simulink model "IntModelY1_20212r"  (R2022b)
settings: Solver=VariableStepAuto  StartTime=0.0  StopTime=inf  RelTol=1e-3
model workspace (MAT data in the model file):
  firstWarning = 1
  originalScenarioChecksum = '114339432DE22364D47BB28FC96DC10C'
undefined symbols (not defined in the file or in its folder): Acceleration, ActorID, AngularVelocity, curvature, curvatureAhd, DefaultGear, DEND_B, DEND_S, DEND_T, direction, driving, gradbp, L, LF, LR, matlabshared, MAX_BRAKE, MAX_STEER, MAX_TORQUE, MCAR, MIN_BRAKE, MIN_STEER, MIN_TORQUE, NUMD_B, NUMD_S, NUMD_T, Pitch, Position, psi_o, R, Roll, RRdamp, SceneInfo, session, sigbuilder_block, STEER_RATIO, stopSign_ID, Tdead, thetaRefs, TL_ID, TrackWidth, Ts, ts, Vdead, Velocity, WB, X_o, xRef2s, Y_o, Yaw, yRef2s
libraries: drivingscenarioandsensors x8, simulink x3, drivingvehiclecontroller x2, trackingutilitieslib x2, robotalgslib x1, mpcadaslib x1, drivinglib x1, simulink_extras x1, autolibshared x1, vehdynlibviscommon x1, vehdynlibsteering x1
(part 2 of 3)

== system IntModelY1_20212r/Environment & Data/Sensors & Perception/Tracking ==
  Detections : Inport
  Camera : drivingscenarioandsensors/Vision Detection Generator  SensorIndex=1  DetectorOutput=Objects only  UpdateInterval=0.01  LaneUpdateInterval=0.1  SensorLocation=[1.9 0]  Height=1.1  Yaw=0  Pitch=1  Roll=0  BusNameSource=Auto  BusName=BusObjectDetections  BusName2Source=Auto  BusName2=BusLaneDetections  MaxNumDetectionsSource=Property  MaxNumDetections=10  MaxNumLanesSource=Property  MaxNumLanes=30  DetectionCoordinates=Ego Cartesian  SimulateUsing=Interpreted execution  MaxRange=150  BoundingBoxAccuracy=5  ProcessNoiseIntensity=5  MaxSpeed=100  MaxAllowedOcclusion=0.5  MinObjectImageSize=[2 2]  DetectionProbability=0.9  FalsePositivesPerImage=0.1  MinLaneImageSize=[20 3]  LaneBoundaryAccuracy=3  HasNoise=on  InitialSeedSource=Repeatable  InitialSeed=0  UsedSeed=0  ActorProfilesSource=From Scenario Reader block  ActorProfilesParameters=driving.internal.ActorProfilesParameters  ActorProfilesExpression=[struct('ActorID',1,'ClassID',1,'Length',4.7,'Width',1.8,'Height',1.4,'OriginOffset',[-1.35 0 0],'MeshVertices',[3.7 0.9 0.857439446366782;3.7 -0.9 0.857439446366782;3.7 -0.9 0.314878892733564;3.7 0.9 0.314878892733564;3.7 0.9 0.857439446366782;2.525 0.9 0.993079584775086;2.525 -0.9 0.993079584775086;3.7 -0.9 0.857439446366782;1.82 0.72 1.4;0.41 0.72 1.4;0.41 -0.72 1.4;1.82 -0.72 1.4;-0.295 0.9 0.993079584775086;-1 0.9 0.857439446366782;-1 -0.9 0.857439446366782;-0.295 -0.9 0.993079584775086;3.7 0.9 0.857439446366782;3.7 0.9 0.314878892733564;2.525 0.9 0.314878892733564;2.525 0.9 0.993079584775086;2.525 0.9 0.993079584775086;2.525 0.9 0.314878892733564;-0.295 0.9 0.314878892733564;-0.295 0.9 0.993079584775086;-0.295 0.9 0.993079584775086;-0.295 0.9 0.314878892733564;-1 0.9 0.355570934256055;-1 0.9 0.857439446366782;2.525 0.9 0.993079584775086;-0.295 0.9 0.993079584775086;0.41 0.72 1.4;1.82 0.72 1.4;3.7 -0.9 0.857439446366782;3.7 -0.9 0.314878892733564;2.525 -0.9 0.314878892733564;2.525 -0.9 0.993079584775086;2.525 -0.9 0.993079584775086;2.525 -0.9 0.314878892733564;-0.295 -0.9 0.314878892733564;-0.295 -0.9 0.993079584775086;-0.295 -0.9 0.993079584775086;-0.295 -0.9 0.314878892733564;-1 -0.9 0.355570934256055;-1 -0.9 0.857439446366782;2.525 -0.9 0.993079584775086;-0.295 -0.9 0.993079584775086;0.41 -0.72 1.4;1.82 -0.72 1.4;-0.295 0.9 0.993079584775086;-0.295 -0.9 0.993079584775086;0.41 -0.72 1.4;0.41 0.72 1.4;2.525 -0.9 0.993079584775086;1.82 -0.72 1.4;1.82 0.72 1.4;2.525 0.9 0.993079584775086;-1 0.9 0.857439446366782;-1 0.9 0.355570934256055;-1 -0.9 0.355570934256055;-1 -0.9 0.857439446366782;3.7 0.9 0.314878892733564;3.7 -0.9 0.314878892733564;-0.295 -0.9 0.314878892733564;-0.295 0.9 0.314878892733564;-0.295 0.9 0.314878892733564;-1 0.9 0.355570934256055;-1 -0.9 0.355570934256055;-0.295 -0.9 0.314878892733564;0 -0.63 0;0 -0.87 0;0.191030206995054 -0.63 0.0601365173421445;0.191030206995054 -0.87 0.0601365173421445;0.309093367795925 -0.63 0.217575963708927;0.309093367795925 -0.87 0.217575963708927;0.309093367795925 -0.63 0.412181821758201;0.309093367795925 -0.87 0.412181821758201;0.191030206995054 -0.63 0.569621268124983;0.191030206995054 -0.87 0.569621268124983;0 -0.63 0.629757785467128;0 -0.87 0.629757785467128;-0.191030206995054 -0.63 0.569621268124983;-0.191030206995054 -0.87 0.569621268124983;-0.309093367795925 -0.63 0.412181821758201;-0.309093367795925 -0.87 0.412181821758201;-0.309093367795925 -0.63 0.217575963708927;-0.309093367795925 -0.87 0.217575963708927;-0.191030206995054 -0.63 0.0601365173421445;-0.191030206995054 -0.87 0.0601365173421445;0 -0.63 0;0 -0.87 0;0 -0.63 0;0.191030206995054 -0.63 0.0601365173421445;0.309093367795925 -0.63 0.217575963708927;0.309093367795925 -0.63 0.412181821758201;0.191030206995054 -0.63 0.569621268124983;0 -0.63 0.629757785467128;-0.191030206995054 -0.63 0.569621268124983;-0.309093367795925 -0.63 0.412181821758201;-0.309093367795925 -0.63 0.217575963708927;-0.191030206995054 -0.63 0.0601365173421445;0 -0.87 0;0.191030206995054 -0.87 0.0601365173421445;0.309093367795925 -0.87 0.217575963708927;0.309093367795925 -0.87 0.412181821758201;0.191030206995054 -0.87 0.569621268124983;0 -0.87 0.629757785467128;-0.191030206995054 -0.87 0.569621268124983;-0.309093367795925 -0.87 0.412181821758201;-0.309093367795925 -0.87 0.217575963708927;-0.191030206995054 -0.87 0.0601365173421445;0 0.87 0;0 0.63 0;0.191030206995054 0.87 0.0601365173421445;0.191030206995054 0.63 0.0601365173421445;0.309093367795925 0.87 0.217575963708927;0.309093367795925 0.63 0.217575963708927;0.309093367795925 0.87 0.412181821758201;0.309093367795925 0.63 0.412181821758201;0.191030206995054 0.87 0.569621268124983;0.191030206995054 0.63 0.569621268124983;0 0.87 0.629757785467128;0 0.63 0.629757785467128;-0.191030206995054 0.87 0.569621268124983;-0.191030206995054 0.63 0.569621268124983;-0.309093367795925 0.87 0.412181821758201;-0.309093367795925 0.63 0.412181821758201;-0.309093367795925 0.87 0.217575963708927;-0.309093367795925 0.63 0.217575963708927;-0.191030206995054 0.87 0.0601365173421445;-0.191030206995054 0.63 0.0601365173421445;0 ...(+3718 chars)],'MeshFaces',[1 2 3;3 4 1;5 6 7;7 8 5;9 10 11;11 12 9;13 14 15;15 16 13;17 18 19;19 20 17;21 22 23;23 24 21;25 26 27;27 28 25;29 30 31;31 32 29;33 34 35;35 36 33;37 38 39;39 40 37;41 42 43;43 44 41;45 46 47;47 48 45;49 50 51;51 52 49;53 54 55;55 56 53;57 58 59;59 60 57;61 62 63;63 64 61;65 66 67;67 68 65;69 71 72;72 70 69;71 73 74;74 72 71;73 75 76;76 74 73;75 77 78;78 76 75;77 79 80;80 78 77;79 81 82;82 80 79;81 83 84;84 82 81;83 85 86;86 84 83;85 87 88;88 86 85;87 89 90;90 88 87;91 92 93;91 93 94;91 94 95;91 95 96;91 96 97;91 97 98;91 98 99;91 99 100;101 102 103;101 103 104;101 104 105;101 105 106;101 106 107;101 107 108;101 108 109;101 109 110;111 113 114;114 112 111;113 115 116;116 114 113;115 117 118;118 116 115;117 119 120;120 118 117;119 121 122;122 120 119;121 123 124;124 122 121;123 125 126;126 124 123;125 127 128;128 126 125;127 129 130;130 128 127;129 131 132;132 130 129;133 134 135;133 135 136;133 136 137;133 137 138;133 138 139;133 139 140;133 140 141;133 141 142;143 144 145;143 145 146;143 146 147;143 147 148;143 148 149;143 149 150;143 150 151;143 151 152;153 155 156;156 154 153;155 157 158;158 156 155;157 159 160;160 158 157;159 161 162;162 160 159;161 163 164;164 162 161;163 165 166;166 164 163;165 167 168;168 166 165;167 169 170;170 168 167;169 171 172;172 170 169;171 173 174;174 172 171;175 176 177;175 177 178;175 178 179;175 179 180;175 180 181;175 181 182;175 182 183;175 183 184;185 186 187;185 187 188;185 188 189;185 189 190;185 190 191;185 191 192;185 192 193;185 193 194;195 197 198;198 196 195;197 199 200;200 198 197;199 201 202;202 200 199;201 203 204;204 202 201;203 205 206;206 204 203;205 207 208;208 206 205;207 209 210;210 208 207;209 211 212;212 210 209;211 213 214;214 212 211;213 215 216;216 214 213;217 218 219;217 219 220;217 220 221;217 221 222;217 222 223;217 223 224;217 224 225;217 225 226;227 228 229;227 229 230;227 230 231;227 231 232;227 232 233;227 233 234;227 234 235;227 235 236],'RCSPattern',[10 10;10 10],'RCSAzimuthAngles',[-180 180],'RCSElevationAngles',[-90 90]); struct('ActorID',2,'ClassID',7,'Length',0.7,'Width',0.2,'Height',0.1,'OriginOffset',[0 0 0],'MeshVertices',[0.35 -0.1 0.1;0.35 0.1 0.1;-0.35 0.1 0.1;-0.35 -0.1 0.1;0.35 -0.1 0;0.35 0.1 0;-0.35 0.1 0;-0.35 -0.1 0],'MeshFaces',[6 2 1;1 5 6;8 4 3;3 7 8;6 7 3;3 2 6;5 1 4;4 8 5;4 1 2;2 3 4;7 6 5;5 8 7],'RCSPattern',[10 10;10 10],'RCSAzimuthAngles',[-180 180],'RCSElevationAngles',[-90 90])]  Intrinsics=driving.internal.cameraIntrinsics('FocalLength',[400 800],'PrincipalPoint',[320 240],'ImageSize',[480 640],'RadialDistortion',[0 0],'TangentialDistortion',[0 0],'Skew',0)
  Detection Concatenation : trackingutilitieslib/Detection Concatenation  NumInputs=2  BusNameSource=Property  BusName=Detections  SimulateUsing=Interpreted execution
  Multi-Object Tracker : drivinglib/Multi-Object Tracker  TrackerIndex=uint32( 0 )  FilterInitializationFcn=helperInitSimulinkDemoFilter  AssignmentThreshold=50  ConfirmationThreshold=[ 2, 3 ]  DeletionThreshold=[ 5, 5 ]  MaxNumTracks=20  MaxNumSensors=20  OOSMHandling=Neglect  StateParametersSimulink=struct  HasStateParametersInput=off  TimeInputSource=Auto  HasCostMatrixInput=off  HasDetectableTrackIDsInput=off  BusNameSource=Auto  BusName=BusMultiObjectTracker  TentativeTracksOutputPort=off  AllTracksOutputPort=off  SimulateUsing=Interpreted execution
  Radar Detection Generator : drivingscenarioandsensors/Radar Detection Generator  SensorIndex=2  UpdateInterval=0.01  SensorLocation=[ 1.5, 0 ]  Height=0.2  Yaw=0  Pitch=0  Roll=0  BusNameSource=Auto  BusName=BusRadarDetectionGenerator  MaxNumDetectionsSource=Property  MaxNumDetections=50  DetectionCoordinates=Ego Cartesian  SimulateUsing=Interpreted execution  AzimuthResolution=4  ElevationResolution=10  RangeResolution=2.5  RangeRateResolution=0.5  AzimuthBiasFraction=0.1  ElevationBiasFraction=0.1  RangeBiasFraction=0.05  RangeRateBiasFraction=0.05  FieldOfView=[ 60, 5 ]  MaxRange=150  RangeRateLimits=[ -100, 100 ]  DetectionProbability=0.9  FalseAlarmRate=1e-6  ReferenceRange=100  ReferenceRCS=0  HasElevation=off  HasRangeRate=on  HasNoise=on  HasFalseAlarms=on  HasOcclusion=on  InitialSeedSource=Repeatable  InitialSeed=0  UsedSeed=matlabshared.tracking.internal.SimulinkUtilities.seedManager(gcb)  ActorProfilesSource=Parameters  ActorProfilesParameters=driving.internal.ActorProfilesRadarParameters  ActorProfilesExpression=struct( 'ClassID', 0, 'Length', 4.7, 'Width', 1.8, 'Height', 1.4, 'OriginOffset', [ -1.35, 0, 0 ], 'RCSPattern', [ 10, 10; 10, 10 ], 'RCSAzimuthAngles', [ -180, 180 ], 'RCSElevationAngles', [ -90, 90 ] )
  Subsystem1 : Subsystem  Commented=on
  Confirmed_Tracks : Outport
  wires:
  Camera/1 -> Detection Concatenation/1  "Camera Detections"
  Radar Detection Generator/1 -> Detection Concatenation/2  "Lidar Detections"
  Detections/1 -> Radar Detection Generator/1, Camera/1
  Detection Concatenation/1 -> Multi-Object Tracker/1
  Multi-Object Tracker/1 -> Confirmed_Tracks/1

== system IntModelY1_20212r/Environment & Data/Visualisation & Data/Lights and Signs ID ==
  Constant : Constant  Value=TL_ID
  Constant1 : Constant  Value=stopSign_ID
  TL : Outport
  Stop_Sign : Outport  Port=2
  wires:
  Constant/1 -> TL/1
  Constant1/1 -> Stop_Sign/1

== system IntModelY1_20212r/Environment & Data/Visualisation & Data/Positions and States  ==
  note: Stop Sign positon
  note: Traffic Light Position and State
  <Actors> : Inport
  TL_id : Inport  Port=2
  ss_State : Inport  Port=3
  MATLAB Function1 : MATLAB Function  TreatAsAtomicUnit=on
  MATLAB Function2 : MATLAB Function  TreatAsAtomicUnit=on
  Traffic Light Sensor : Subsystem  mask{TrafficLightSensorModeSelection=Cycle}
      mask prompts: TrafficLightSensorModeSelection "Traffic Light Sensor Mode:"
      mask TypeOptions TrafficLightSensorModeSelection: Steady Green | Steady Red | Cycle
      mask DialogControl DescTextVar Prompt: Simulate a traffic light sensor.
  TL_poses : Outport
  ss_poses : Outport  Port=2
  wires:
  <Actors>/1 -> MATLAB Function2/1(Actors), MATLAB Function1/1(Actors)
  ss_State/1 -> MATLAB Function2/2(ss_State)
  TL_id/1 -> Traffic Light Sensor/1(TL_id)
  Traffic Light Sensor/1(TL_State) -> MATLAB Function1/2(TL_State)  "TL_State"
  MATLAB Function2/1(ss_poses) -> ss_poses/1
  MATLAB Function1/1(TL_poses) -> TL_poses/1

== system IntModelY1_20212r/Environment & Data/Visualisation & Data/Visualization ==
  note: Visualization
  TL1_poses : Inport
  Actors : Inport  Port=2
  EgoInfo : Inport  Port=3
  ss1_poses : Inport  Port=4
  Visualization : MATLABSystem  System=TL_vis
      mask Type: TL_vis
      mask Display:
      | disp('TL_vis');
      | port_label('input',1,'TL');
      | port_label('input',2,'TargetPoses');
      | port_label('input',3,'EgoInfo');
      | port_label('input',4,'SS');
  wires:
  EgoInfo/1 -> Visualization/3
  Actors/1 -> Visualization/2  "target_vehicle_poses"
  TL1_poses/1 -> Visualization/1
  ss1_poses/1 -> Visualization/4

== system IntModelY1_20212r/Reference Data/Theta/thetaBlocks ==
  note: theta calculated from Simulink blocks
  y : Inport
  x : Inport  Port=2
  dis : Inport  Port=3
  Atan2 : Trigonometry  Operator=atan2  ApproximationMethod=CORDIC
  Difference : simulink/Discrete/Difference  ICPrevInput=0.0  OutMin=[]  OutMax=[]  OutDataType=fixdt(1, 16)  OutScaling=2^-10  DoSatur=off
  Difference1 : simulink/Discrete/Difference  ICPrevInput=0.0  OutMin=[]  OutMax=[]  OutDataType=fixdt(1, 16)  OutScaling=2^-10  DoSatur=off
  IC : InitialCondition  Value=psi_o
  Radians to Degrees : simulink_extras/Transformations/Radians to Degrees
  Terminator : Terminator
  theta : Outport
  wires:
  IC/1 -> Radians to Degrees/1
  Atan2/1 -> IC/1
  dis/1 -> Terminator/1
  x/1 -> Difference1/1
  y/1 -> Difference/1
  Radians to Degrees/1 -> theta/1
  Difference/1 -> Atan2/1
  Difference1/1 -> Atan2/2

== system IntModelY1_20212r/Reference Data/Theta/thetaLt ==
  note: Check out the script "setUpModel" to understand how we have calculated theta
  note: theta based on lookup table
  y : Inport
  x : Inport  Port=2
  dis : Inport  Port=3
  Terminator : Terminator
  Terminator1 : Terminator
  Theta Ref : Lookup_n-D  NumberOfTableDimensions=1  BreakpointsForDimension1=gradbp  Table=thetaRefs  InternalRulePriority=Speed  RndMeth=Simplest
  theta : Outport
  wires:
  Theta Ref/1 -> theta/1
  dis/1 -> Theta Ref/1
  x/1 -> Terminator1/1
  y/1 -> Terminator/1

== system IntModelY1_20212r/Vehicle Dynamics/Subsystem/Signal Builder ==
  Demux : Demux  Tag=STV Demux  Outputs=3
      settings: DisplayOption=none
  FromWs : FromWorkspace  Tag=STV FromWs  VariableName=tuvar
      SigBuilderData=|
      | common.afterFinalStr = 'Extrapolate'
      | common.sampleTime = 0
      | dataSet.timeRange = [0 3.5]
      | dataSet.name = 'DriveAndTurn'
      | sbobj.Groups.Name = 'DriveAndTurn'
      | sbobj.Groups.Signals(1).Name = 'Normalized Torque'
      | sbobj.Groups.Signals(1).XData = [0 1 1 2 2 3.5]
      | sbobj.Groups.Signals(1).YData = [1 1 0 0 1 1]
      | sbobj.Groups.Signals(2).Name = 'Normalized Brake'
      | sbobj.Groups.Signals(2).XData = [0 1 1 2 2 3.5]
      | sbobj.Groups.Signals(2).YData = [0 0 1 1 0 0]
      | sbobj.Groups.Signals(3).Name = 'Normalized Steer'
      | sbobj.Groups.Signals(3).XData = [0 0.5 0.6 1.02 1.02 2 2.5 3 3.5]
      | sbobj.Groups.Signals(3).YData = [-0.02 -0.02 -0.02 -0.3 -1.02 -0.92 -0.34 0.14 0.22]
      | sbobj.Groups.TimeRange = [0 3.5]
  Normalized Torque : Outport  Tag=STV Outport
  Normalized Brake : Outport  Tag=STV Outport  Port=2
  Normalized Steer : Outport  Tag=STV Outport  Port=3
  wires:
  FromWs/1 -> Demux/1
  Demux/1 -> Normalized Torque/1
  Demux/2 -> Normalized Brake/1
  Demux/3 -> Normalized Steer/1

== system IntModelY1_20212r/Vehicle Dynamics/VehicleDynamics/Vehicle XY Plotter ==
  VehFdbk : Inport
  VehFdbk1 : Inport  Port=2
  Bus Selector1 : BusSelector  OutputSignals=InertFrm.Cg.Ang.phi,InertFrm.Cg.Ang.theta,InertFrm.Cg.Ang.psi  OutputAsBus=on
  Bus Selector3 : BusSelector  OutputSignals=InertFrm.Geom.Disp.X,InertFrm.Geom.Disp.Y,InertFrm.Geom.Disp.Z  OutputAsBus=on
  Bus Selector4 : BusSelector  OutputSignals=InertFrm.Cg.Vel.Xdot,InertFrm.Cg.Vel.Ydot  OutputAsBus=on
  Bus to Vector : BusToVector
  Bus to Vector1 : BusToVector
  Bus to Vector2 : BusToVector
  Constant4 : Constant  Value=0
  Ground : Ground
  Rate Transition{1..2,5..6} (4 alike) : RateTransition  OutPortSampleTime=pltDT
  Vector Concatenate : Concatenate
  Vector Concatenate1 : Concatenate  NumInputs=4
  Vehicle XY Plotter : vehdynlibviscommon/Vehicle XY Plotter  w=w  a=a  b=b  figBorder=2000  bufferSize=bufferSize  extStats=off  extTireF=off
  wires:
  Bus to Vector2/1 -> Rate Transition1/1  "InertCGDisp"
  Rate Transition5/1 -> Vehicle XY Plotter/1
  Bus Selector4/1 -> Bus to Vector1/1
  Rate Transition1/1 -> Vehicle XY Plotter/2
  Rate Transition6/1 -> Vehicle XY Plotter/3
  Vector Concatenate/1 -> Rate Transition6/1  "InertCGVel"
  Bus Selector1/1 -> Bus to Vector2/1
  Bus to Vector/1 -> Rate Transition5/1  "InertCGDisp"
  Bus Selector3/1 -> Bus to Vector/1
  Bus to Vector1/1 -> Vector Concatenate/1
  Ground/1 -> Vector Concatenate/2
  VehFdbk/1 -> Bus Selector1/1, Bus Selector4/1, Bus Selector3/1
  Rate Transition2/1 -> Vehicle XY Plotter/4
  Constant4/1 -> Vector Concatenate1/4, Vector Concatenate1/3
  VehFdbk1/1 -> Vector Concatenate1/2, Vector Concatenate1/1  "delta"
  Vector Concatenate1/1 -> Rate Transition2/1  "delta"

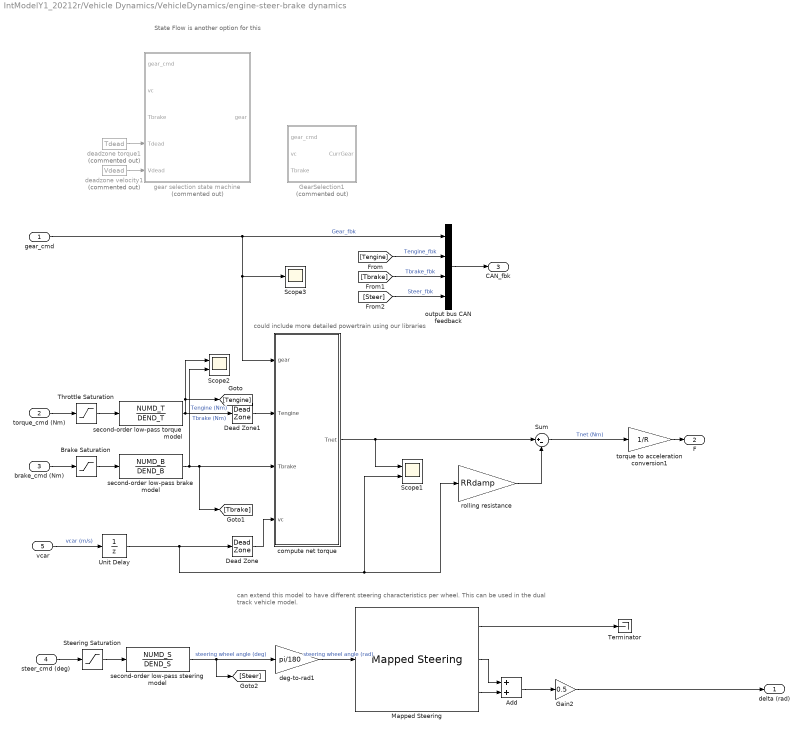
== system IntModelY1_20212r/Vehicle Dynamics/VehicleDynamics/engine-steer-brake dynamics ==
  note: State Flow is another option for this
  note: could include more detailed powertrain using our libraries
  note: can extend this model to have different steering characteristics per wheel. This can be used in the dual track vehicle model.
  gear_cmd : Inport
  torque_cmd (Nm) : Inport  Port=2
  brake_cmd (Nm) : Inport  Port=3
  steer_cmd (deg) : Inport  Port=4
  vcar : Inport  Port=5
  Add : Sum
  Brake Saturation : Saturate  UpperLimit=MAX_BRAKE  LowerLimit=MIN_BRAKE
  Dead Zone : DeadZone  LowerValue=-Vdead  UpperValue=Vdead
  Dead Zone1 : DeadZone  LowerValue=-Tdead  UpperValue=Tdead
  Gain2 : Gain  Gain=0.5
  GearSelection1 : Stateflow chart  Commented=on  TreatAsAtomicUnit=on  SystemSampleTime=ts
      settings: PortSchema="{\"entries\":[{\"content\":{\"sides\":[{\"content\":{\"connectorIds\":[\"In3\",\"In2\",\"In1\"]},\"type\":\"ConnectorPlacement.EquallySpacedRectSide\",\"uuid\":\"465e5722-891f-481b-b3b6-2b8339e8e743\"},{\"content\":{\"connectorIds\":[\"Out1\"],\"side\":\"RIGHT\"},\"type\":\"ConnectorPlacement.EquallySpacedRectSide\",\"uuid\":\"28ef13cd-41d9-4e2e-8cd9-9157abf573a9\"},{\"content\":{\"connectorIds\":[],\"side\":\"TOP\"},\"type\":\"ConnectorPlacement.EquallySpacedRectSide\",\"uuid\":\"44f19923-60ae-466f-ad2a-756f1033b52e\"},{\"content\":{\"connectorIds\":[],\"side\":\"HIDDEN\"},\"type\":\"ConnectorPlacement.EquallySpacedRectSide\",\"uuid\":\"d5a146f0-4328-42be-94e3-09f51634e7da\"}]},\"type\":\"ConnectorPlacement.EquallySpacedConnector\",\"uuid\":\"14e271af-3da2-4f7d-9688-fcc3c9792006\"}],\"packageUris\":[\"http://schema.mathworks.com/mf0/Connector/R2020b\"],\"version\":\"1.0\"}"
  Mapped Steering : vehdynlibsteering/Mapped Steering  SpdDpd=off  IndexType=Steering wheel angle  GrType=Constant  StrgAngBpts=[-1.5*pi 1.5*pi]  RackDispBpts=[-40 -19.2 -4.53 4.53 19.2 40]  Gr=8.28*2*pi  GrTbl=[9.87 9.87 7.16 7.16 9.87 9.87]*2*pi  WhlLftTbl=[-1.5*pi 1.5*pi]*STEER_RATIO  WhlRghtTbl=[-1.5*pi 1.5*pi]*STEER_RATIO  VehSpdBpts=[-1 1]  SpdFctTbl=[1 1]  aMode=2
  Scope1 : Scope  NumInputPorts=2
  Scope2 : Scope  NumInputPorts=2
  Scope3 : Scope
  Steering Saturation : Saturate  UpperLimit=MAX_STEER  LowerLimit=MIN_STEER
  Sum : Sum  Inputs=|+-
  Terminator : Terminator
  Throttle Saturation : Saturate  UpperLimit=MAX_TORQUE  LowerLimit=MIN_TORQUE
  Unit Delay : UnitDelay  SampleTime=-1  HasFrameUpgradeWarning=on
  compute net torque : MATLAB Function  TreatAsAtomicUnit=on  SystemSampleTime=ts
  deadzone torque1 : Constant  Commented=on  Value=Tdead  SampleTime=ts
  deadzone velocity1 : Constant  Commented=on  Value=Vdead  SampleTime=ts
  deg-to-rad1 : Gain  Gain=pi/180
  gear selection state machine : MATLAB Function  Commented=on  TreatAsAtomicUnit=on  SystemSampleTime=ts
  output bus CAN feedback : BusCreator  Inputs=4
  rolling resistance : Gain  Gain=RRdamp
  second-order low-pass brake model : DiscreteTransferFcn  Numerator=NUMD_B  Denominator=DEND_B  SampleTime=ts
  second-order low-pass steering model : DiscreteTransferFcn  Numerator=NUMD_S  Denominator=DEND_S  SampleTime=ts
  second-order low-pass torque model : DiscreteTransferFcn  Numerator=NUMD_T  Denominator=DEND_T  SampleTime=ts
  torque to acceleration conversion1 : Gain  Gain=1/R
  delta (rad) : Outport  VectorParamsAs1DForOutWhenUnconnected=off
  F : Outport  Port=2  VectorParamsAs1DForOutWhenUnconnected=off
  CAN_fbk : Outport  Port=3  VectorParamsAs1DForOutWhenUnconnected=off
  wires:
  steer_cmd (deg)/1 -> Steering Saturation/1
  torque_cmd (Nm)/1 -> Throttle Saturation/1
  brake_cmd (Nm)/1 -> Brake Saturation/1
  second-order low-pass steering model/1 -> deg-to-rad1/1, [Steer]  "steering wheel angle (deg)"
  Throttle Saturation/1 -> second-order low-pass torque model/1
  Brake Saturation/1 -> second-order low-pass brake model/1
  Steering Saturation/1 -> second-order low-pass steering model/1
  vcar/1 -> Unit Delay/1  "vcar (m/s)"
  second-order low-pass brake model/1 -> [Tbrake], compute net torque/3(Tbrake), Scope2/2  "Tbrake (Nm)"
  second-order low-pass torque model/1 -> Dead Zone1/1, [Tengine], Scope2/1  "Tengine (Nm)"
  compute net torque/1(Tnet) -> Scope1/1, Sum/1
  rolling resistance/1 -> Sum/2
  deadzone velocity1/1 -> gear selection state machine/5(Vdead)
  deadzone torque1/1 -> gear selection state machine/4(Tdead)
  gear_cmd/1 -> output bus CAN feedback/1, Scope3/1, compute net torque/1(gear)  "Gear_fbk"
  output bus CAN feedback/1 -> CAN_fbk/1
  [Tengine] -> output bus CAN feedback/2  "Tengine_fbk"
  [Tbrake] -> output bus CAN feedback/3  "Tbrake_fbk"
  [Steer] -> output bus CAN feedback/4  "Steer_fbk"
  Mapped Steering/2 -> Add/1
  Mapped Steering/3 -> Add/2
  Add/1 -> Gain2/1
  torque to acceleration conversion1/1 -> F/1
  Mapped Steering/1 -> Terminator/1
  deg-to-rad1/1 -> Mapped Steering/1  "steering wheel angle (rad)"
  Sum/1 -> torque to acceleration conversion1/1  "Tnet (Nm)"
  Dead Zone/1 -> compute net torque/4(vc)
  Dead Zone1/1 -> compute net torque/2(Tengine)
  Unit Delay/1 -> Scope1/2, rolling resistance/1, Dead Zone/1
  Gain2/1 -> delta (rad)/1

== system IntModelY1_20212r/Controllers/Lateral Controllers/Pure Pursuit Controller1/Wheel Steering Angle Formulation ==
  alpha : Inport
  Bicycle length : Constant  Value=L
  Constant : Constant  Value=2
  Divide : Product  Inputs=*/
  Lookahead distance : Constant  Value=ld
  Product : Product
  Product1 : Product
  Sine Wave : Sin  TimeSource=Use external signal  SampleTime=0
  Trigonometric Function : Trigonometry  Operator=atan
  Al : Outport
  wires:
  Sine Wave/1 -> Product1/2
  Bicycle length/1 -> Product/2
  Constant/1 -> Product/1
  Product1/1 -> Divide/1
  Product/1 -> Product1/1
  Divide/1 -> Trigonometric Function/1
  Trigonometric Function/1 -> Al/1
  alpha/1 -> Sine Wave/1
  Lookahead distance/1 -> Divide/2

== system IntModelY1_20212r/Controllers/Subsystem3/Subsystem1/Subsystem2 ==
  acc_cmd : Inport
  decc_cmd : Inport  Port=2
  Subsystem : Subsystem
  Subsystem1 : Subsystem
  T_eng_cmd : Outport
  brake_cmd : Outport  Port=2
  wires:
  acc_cmd/1 -> Subsystem/1(acc_cmd)
  Subsystem/1(T_eng_cmd) -> T_eng_cmd/1
  decc_cmd/1 -> Subsystem1/1(decc_cmd)
  Subsystem1/1(T_brake_cmd) -> brake_cmd/1

== system IntModelY1_20212r/Controllers/Subsystem3/Subsystem2/Subsystem2 ==
  acc_cmd : Inport
  decc_cmd : Inport  Port=2
  Subsystem : Subsystem
  Subsystem1 : Subsystem
  T_eng_cmd : Outport
  brake_cmd : Outport  Port=2
  wires:
  acc_cmd/1 -> Subsystem/1(acc_cmd)
  Subsystem/1(T_eng_cmd) -> T_eng_cmd/1
  decc_cmd/1 -> Subsystem1/1(decc_cmd)
  Subsystem1/1(T_brake_cmd) -> brake_cmd/1

== system IntModelY1_20212r/Environment & Data/Sensors & Perception/Tracking/Subsystem1 ==
  In2 : Inport
  EgoV : Inport  Port=2
  Camera : drivingscenarioandsensors/Vision Detection Generator  SensorIndex=1  DetectorOutput=Objects only  UpdateInterval=0.1  LaneUpdateInterval=0.1  SensorLocation=[1.9 0]  Height=1.1  Yaw=0  Pitch=1  Roll=0  BusNameSource=Auto  BusName=BusObjectDetections  BusName2Source=Auto  BusName2=BusLaneDetections  MaxNumDetectionsSource=Property  MaxNumDetections=10  MaxNumLanesSource=Property  MaxNumLanes=30  DetectionCoordinates=Ego Cartesian  SimulateUsing=Interpreted execution  MaxRange=150  BoundingBoxAccuracy=5  ProcessNoiseIntensity=5  MaxSpeed=100  MaxAllowedOcclusion=0.5  MinObjectImageSize=[5 5]  DetectionProbability=0.9  FalsePositivesPerImage=0.1  MinLaneImageSize=[20 3]  LaneBoundaryAccuracy=3  HasNoise=on  InitialSeedSource=Repeatable  InitialSeed=0  UsedSeed=0  ActorProfilesSource=From Scenario Reader block  ActorProfilesParameters=driving.internal.ActorProfilesParameters  ActorProfilesExpression=[struct('ActorID',1,'ClassID',1,'Length',4.7,'Width',1.8,'Height',1.4,'OriginOffset',[-1.35 0 0],'MeshVertices',[3.7 0.9 0.857439446366782;3.7 -0.9 0.857439446366782;3.7 -0.9 0.314878892733564;3.7 0.9 0.314878892733564;3.7 0.9 0.857439446366782;2.525 0.9 0.993079584775086;2.525 -0.9 0.993079584775086;3.7 -0.9 0.857439446366782;1.82 0.72 1.4;0.41 0.72 1.4;0.41 -0.72 1.4;1.82 -0.72 1.4;-0.295 0.9 0.993079584775086;-1 0.9 0.857439446366782;-1 -0.9 0.857439446366782;-0.295 -0.9 0.993079584775086;3.7 0.9 0.857439446366782;3.7 0.9 0.314878892733564;2.525 0.9 0.314878892733564;2.525 0.9 0.993079584775086;2.525 0.9 0.993079584775086;2.525 0.9 0.314878892733564;-0.295 0.9 0.314878892733564;-0.295 0.9 0.993079584775086;-0.295 0.9 0.993079584775086;-0.295 0.9 0.314878892733564;-1 0.9 0.355570934256055;-1 0.9 0.857439446366782;2.525 0.9 0.993079584775086;-0.295 0.9 0.993079584775086;0.41 0.72 1.4;1.82 0.72 1.4;3.7 -0.9 0.857439446366782;3.7 -0.9 0.314878892733564;2.525 -0.9 0.314878892733564;2.525 -0.9 0.993079584775086;2.525 -0.9 0.993079584775086;2.525 -0.9 0.314878892733564;-0.295 -0.9 0.314878892733564;-0.295 -0.9 0.993079584775086;-0.295 -0.9 0.993079584775086;-0.295 -0.9 0.314878892733564;-1 -0.9 0.355570934256055;-1 -0.9 0.857439446366782;2.525 -0.9 0.993079584775086;-0.295 -0.9 0.993079584775086;0.41 -0.72 1.4;1.82 -0.72 1.4;-0.295 0.9 0.993079584775086;-0.295 -0.9 0.993079584775086;0.41 -0.72 1.4;0.41 0.72 1.4;2.525 -0.9 0.993079584775086;1.82 -0.72 1.4;1.82 0.72 1.4;2.525 0.9 0.993079584775086;-1 0.9 0.857439446366782;-1 0.9 0.355570934256055;-1 -0.9 0.355570934256055;-1 -0.9 0.857439446366782;3.7 0.9 0.314878892733564;3.7 -0.9 0.314878892733564;-0.295 -0.9 0.314878892733564;-0.295 0.9 0.314878892733564;-0.295 0.9 0.314878892733564;-1 0.9 0.355570934256055;-1 -0.9 0.355570934256055;-0.295 -0.9 0.314878892733564;0 -0.63 0;0 -0.87 0;0.191030206995054 -0.63 0.0601365173421445;0.191030206995054 -0.87 0.0601365173421445;0.309093367795925 -0.63 0.217575963708927;0.309093367795925 -0.87 0.217575963708927;0.309093367795925 -0.63 0.412181821758201;0.309093367795925 -0.87 0.412181821758201;0.191030206995054 -0.63 0.569621268124983;0.191030206995054 -0.87 0.569621268124983;0 -0.63 0.629757785467128;0 -0.87 0.629757785467128;-0.191030206995054 -0.63 0.569621268124983;-0.191030206995054 -0.87 0.569621268124983;-0.309093367795925 -0.63 0.412181821758201;-0.309093367795925 -0.87 0.412181821758201;-0.309093367795925 -0.63 0.217575963708927;-0.309093367795925 -0.87 0.217575963708927;-0.191030206995054 -0.63 0.0601365173421445;-0.191030206995054 -0.87 0.0601365173421445;0 -0.63 0;0 -0.87 0;0 -0.63 0;0.191030206995054 -0.63 0.0601365173421445;0.309093367795925 -0.63 0.217575963708927;0.309093367795925 -0.63 0.412181821758201;0.191030206995054 -0.63 0.569621268124983;0 -0.63 0.629757785467128;-0.191030206995054 -0.63 0.569621268124983;-0.309093367795925 -0.63 0.412181821758201;-0.309093367795925 -0.63 0.217575963708927;-0.191030206995054 -0.63 0.0601365173421445;0 -0.87 0;0.191030206995054 -0.87 0.0601365173421445;0.309093367795925 -0.87 0.217575963708927;0.309093367795925 -0.87 0.412181821758201;0.191030206995054 -0.87 0.569621268124983;0 -0.87 0.629757785467128;-0.191030206995054 -0.87 0.569621268124983;-0.309093367795925 -0.87 0.412181821758201;-0.309093367795925 -0.87 0.217575963708927;-0.191030206995054 -0.87 0.0601365173421445;0 0.87 0;0 0.63 0;0.191030206995054 0.87 0.0601365173421445;0.191030206995054 0.63 0.0601365173421445;0.309093367795925 0.87 0.217575963708927;0.309093367795925 0.63 0.217575963708927;0.309093367795925 0.87 0.412181821758201;0.309093367795925 0.63 0.412181821758201;0.191030206995054 0.87 0.569621268124983;0.191030206995054 0.63 0.569621268124983;0 0.87 0.629757785467128;0 0.63 0.629757785467128;-0.191030206995054 0.87 0.569621268124983;-0.191030206995054 0.63 0.569621268124983;-0.309093367795925 0.87 0.412181821758201;-0.309093367795925 0.63 0.412181821758201;-0.309093367795925 0.87 0.217575963708927;-0.309093367795925 0.63 0.217575963708927;-0.191030206995054 0.87 0.0601365173421445;-0.191030206995054 0.63 0.0601365173421445;0 ...(+3718 chars)],'MeshFaces',[1 2 3;3 4 1;5 6 7;7 8 5;9 10 11;11 12 9;13 14 15;15 16 13;17 18 19;19 20 17;21 22 23;23 24 21;25 26 27;27 28 25;29 30 31;31 32 29;33 34 35;35 36 33;37 38 39;39 40 37;41 42 43;43 44 41;45 46 47;47 48 45;49 50 51;51 52 49;53 54 55;55 56 53;57 58 59;59 60 57;61 62 63;63 64 61;65 66 67;67 68 65;69 71 72;72 70 69;71 73 74;74 72 71;73 75 76;76 74 73;75 77 78;78 76 75;77 79 80;80 78 77;79 81 82;82 80 79;81 83 84;84 82 81;83 85 86;86 84 83;85 87 88;88 86 85;87 89 90;90 88 87;91 92 93;91 93 94;91 94 95;91 95 96;91 96 97;91 97 98;91 98 99;91 99 100;101 102 103;101 103 104;101 104 105;101 105 106;101 106 107;101 107 108;101 108 109;101 109 110;111 113 114;114 112 111;113 115 116;116 114 113;115 117 118;118 116 115;117 119 120;120 118 117;119 121 122;122 120 119;121 123 124;124 122 121;123 125 126;126 124 123;125 127 128;128 126 125;127 129 130;130 128 127;129 131 132;132 130 129;133 134 135;133 135 136;133 136 137;133 137 138;133 138 139;133 139 140;133 140 141;133 141 142;143 144 145;143 145 146;143 146 147;143 147 148;143 148 149;143 149 150;143 150 151;143 151 152;153 155 156;156 154 153;155 157 158;158 156 155;157 159 160;160 158 157;159 161 162;162 160 159;161 163 164;164 162 161;163 165 166;166 164 163;165 167 168;168 166 165;167 169 170;170 168 167;169 171 172;172 170 169;171 173 174;174 172 171;175 176 177;175 177 178;175 178 179;175 179 180;175 180 181;175 181 182;175 182 183;175 183 184;185 186 187;185 187 188;185 188 189;185 189 190;185 190 191;185 191 192;185 192 193;185 193 194;195 197 198;198 196 195;197 199 200;200 198 197;199 201 202;202 200 199;201 203 204;204 202 201;203 205 206;206 204 203;205 207 208;208 206 205;207 209 210;210 208 207;209 211 212;212 210 209;211 213 214;214 212 211;213 215 216;216 214 213;217 218 219;217 219 220;217 220 221;217 221 222;217 222 223;217 223 224;217 224 225;217 225 226;227 228 229;227 229 230;227 230 231;227 231 232;227 232 233;227 233 234;227 234 235;227 235 236],'RCSPattern',[10 10;10 10],'RCSAzimuthAngles',[-180 180],'RCSElevationAngles',[-90 90]); struct('ActorID',2,'ClassID',7,'Length',0.7,'Width',0.2,'Height',0.1,'OriginOffset',[0 0 0],'MeshVertices',[0.35 -0.1 0.1;0.35 0.1 0.1;-0.35 0.1 0.1;-0.35 -0.1 0.1;0.35 -0.1 0;0.35 0.1 0;-0.35 0.1 0;-0.35 -0.1 0],'MeshFaces',[6 2 1;1 5 6;8 4 3;3 7 8;6 7 3;3 2 6;5 1 4;4 8 5;4 1 2;2 3 4;7 6 5;5 8 7],'RCSPattern',[10 10;10 10],'RCSAzimuthAngles',[-180 180],'RCSElevationAngles',[-90 90])]  Intrinsics=driving.internal.cameraIntrinsics('FocalLength',[800 800],'PrincipalPoint',[320 240],'ImageSize',[480 640],'RadialDistortion',[0 0],'TangentialDistortion',[0 0],'Skew',0)
  Detection Concatenation : trackingutilitieslib/Detection Concatenation  NumInputs=3  BusNameSource=Auto  BusName=BusDetectionConcatenation  SimulateUsing=Interpreted execution
  Lidar Point Cloud Generator : drivingscenarioandsensors/Lidar Point Cloud Generator  SensorIndex=2  UpdateInterval=0.1  SensorLocation=[1.5 0]  Height=1.6  Yaw=0  Pitch=0  Roll=0  DetectionCoordinates=Ego Cartesian  HasEgoVehicle=on  EgoVehicleActorID=1  HasRoadsInputPort=on  ActorProfilesSource=From Scenario Reader block  ActorProfilesVariableName=actor_profiles  MaxRange=120  RangeAccuracy=0.002  AzimuthResolution=0.16  ElevationResolution=1.25  AzimuthLimits=[-60 60]  ElevationLimits=[ -20, 20 ]  HasNoise=on
  Lidar Point Cloud Generator1 : drivingscenarioandsensors/Lidar Point Cloud Generator  SensorIndex=3  UpdateInterval=0.1  SensorLocation=[1.5 0]  Height=1.6  Yaw=0  Pitch=0  Roll=0  DetectionCoordinates=Ego Cartesian  HasEgoVehicle=on  EgoVehicleActorID=1  HasRoadsInputPort=on  ActorProfilesSource=From Scenario Reader block  ActorProfilesVariableName=actor_profiles  MaxRange=120  RangeAccuracy=0.002  AzimuthResolution=0.16  ElevationResolution=1.25  AzimuthLimits=[60 180]  ElevationLimits=[ -20, 20 ]  HasNoise=on
  Lidar Point Cloud Generator2 : drivingscenarioandsensors/Lidar Point Cloud Generator  SensorIndex=4  UpdateInterval=0.1  SensorLocation=[1.5 0]  Height=1.6  Yaw=0  Pitch=0  Roll=0  DetectionCoordinates=Ego Cartesian  HasEgoVehicle=on  EgoVehicleActorID=1  HasRoadsInputPort=on  ActorProfilesSource=From Scenario Reader block  ActorProfilesVariableName=actor_profiles  MaxRange=120  RangeAccuracy=0.002  AzimuthResolution=0.16  ElevationResolution=1.25  AzimuthLimits=[-180 -60]  ElevationLimits=[ -20, 20 ]  HasNoise=on
  Camera Detections : Outport
  Radar detections : Outport  Port=2
  wires:
  EgoV/1 -> Lidar Point Cloud Generator1/2, Lidar Point Cloud Generator/2, Lidar Point Cloud Generator2/2
  Lidar Point Cloud Generator1/1 -> Detection Concatenation/2  "Lidar Detections"
  Lidar Point Cloud Generator2/1 -> Detection Concatenation/3  "Lidar Detections"
  Detection Concatenation/1 -> Radar detections/1
  Camera/1 -> Camera Detections/1  "Camera Detections"
  In2/1 -> Camera/1, Lidar Point Cloud Generator/1, Lidar Point Cloud Generator1/1, Lidar Point Cloud Generator2/1
  Lidar Point Cloud Generator/1 -> Detection Concatenation/1  "Lidar Detections"

== system IntModelY1_20212r/Environment & Data/Visualisation & Data/Positions and States /Traffic Light Sensor ==
  note: Traffic Light Sensor
  TL_id : Inport
  Bus Creator : BusCreator  Inputs=2
  LightConfiguration : Constant  Value=TrafficLightSensorModeSelection
  Traffic Light Switching Logic : Stateflow chart  TreatAsAtomicUnit=on
  TL_State : Outport
  wires:
  LightConfiguration/1 -> Traffic Light Switching Logic/1(LightConfig)
  TL_id/1 -> Traffic Light Switching Logic/2(TL_id)
  Bus Creator/1 -> TL_State/1
  Traffic Light Switching Logic/2(trafficLight) -> Bus Creator/1
  Traffic Light Switching Logic/1(TL_ID) -> Bus Creator/2

== system IntModelY1_20212r/Controllers/Subsystem3/Subsystem1/Subsystem2/Subsystem ==
  acc_cmd : Inport
  Constant1 : Constant  Value=MCAR
  Gain : Gain  Gain=1.1*MCAR
  Gain1 : Gain  Gain=1.2*0.3*2/2
  Gain2 : Gain  Gain=0.7*9.81
  Gain4 : Gain  Gain=R/(7.05*0.8)
  Integrator : Integrator  ExternalReset=falling
  Square : Math  Operator=square
  Sum : Sum  Inputs=+++
  T_eng_cmd : Outport
  wires:
  Constant1/1 -> Gain2/1
  Gain/1 -> Sum/3
  Sum/1 -> Gain4/1
  acc_cmd/1 -> Gain/1, Integrator/2, Integrator/1
  Gain2/1 -> Sum/2
  Gain1/1 -> Sum/1  "F_aero"
  Gain4/1 -> T_eng_cmd/1  "T_eng"
  Integrator/1 -> Square/1  "v"
  Square/1 -> Gain1/1

== system IntModelY1_20212r/Controllers/Subsystem3/Subsystem1/Subsystem2/Subsystem1 ==
  decc_cmd : Inport
  Constant1 : Constant  Value=MCAR
  Gain : Gain  Gain=1.1*MCAR
  Gain1 : Gain  Gain=1.2*0.3*2/2
  Gain2 : Gain  Gain=0.7*9.81
  Gain4 : Gain  Gain=-R/(7.05*0.8)
  Integrator : Integrator  ExternalReset=falling
  Square : Math  Operator=square
  Sum : Sum  Inputs=+++
  T_brake_cmd : Outport
  wires:
  Square/1 -> Gain1/1
  Integrator/1 -> Square/1  "v"
  Gain4/1 -> T_brake_cmd/1  "T_eng"
  Gain1/1 -> Sum/1  "F_aero"
  Gain2/1 -> Sum/2
  decc_cmd/1 -> Integrator/2, Integrator/1, Gain/1
  Sum/1 -> Gain4/1
  Gain/1 -> Sum/3
  Constant1/1 -> Gain2/1

== system IntModelY1_20212r/Controllers/Subsystem3/Subsystem2/Subsystem2/Subsystem ==
  acc_cmd : Inport
  Constant1 : Constant  Value=MCAR
  Gain : Gain  Gain=1.1*MCAR
  Gain1 : Gain  Gain=1.2*0.3*2/2
  Gain2 : Gain  Gain=0.7*9.81
  Gain4 : Gain  Gain=R/(7.05*0.8)
  Integrator : Integrator  ExternalReset=falling
  Square : Math  Operator=square
  Sum : Sum  Inputs=+++
  T_eng_cmd : Outport
  wires:
  Constant1/1 -> Gain2/1
  Gain/1 -> Sum/3
  Sum/1 -> Gain4/1
  acc_cmd/1 -> Gain/1, Integrator/2, Integrator/1
  Gain2/1 -> Sum/2
  Gain1/1 -> Sum/1  "F_aero"
  Gain4/1 -> T_eng_cmd/1  "T_eng"
  Integrator/1 -> Square/1  "v"
  Square/1 -> Gain1/1

== system IntModelY1_20212r/Controllers/Subsystem3/Subsystem2/Subsystem2/Subsystem1 ==
  decc_cmd : Inport
  Constant1 : Constant  Value=MCAR
  Gain : Gain  Gain=1.1*MCAR
  Gain1 : Gain  Gain=1.2*0.3*2/2
  Gain2 : Gain  Gain=0.7*9.81
  Gain4 : Gain  Gain=-R/(7.05*0.8)
  Integrator : Integrator  ExternalReset=falling
  Square : Math  Operator=square
  Sum : Sum  Inputs=+++
  T_brake_cmd : Outport
  wires:
  Square/1 -> Gain1/1
  Integrator/1 -> Square/1  "v"
  Gain4/1 -> T_brake_cmd/1  "T_eng"
  Gain1/1 -> Sum/1  "F_aero"
  Gain2/1 -> Sum/2
  decc_cmd/1 -> Integrator/2, Integrator/1, Gain/1
  Sum/1 -> Gain4/1
  Gain/1 -> Sum/3
  Constant1/1 -> Gain2/1

== matlab function IntModelY1_20212r/Environment & Data/Visualisation & Data/Positions and States /MATLAB Function2 ==
  data: Actors input; ss_poses output; ss_State input

function ss_poses = findssposes(Actors, ss_State)

n=length(ss_State);
ss_poses=zeros(n,4);
indices=zeros(n,1);
ID=zeros(length(Actors),1);

for i=1:length(Actors)
 ID(i)=Actors(i).ActorID;
end

indices=find(ismember(ID,ss_State));
if(~isempty(indices))
    
    for i=1:n
        ss_poses(i,:)=([Actors(indices(i)).Position(:)',ss_State(i)]);
    end
end

ss_poses(ss_poses==0)=NaN;






% ss1_poses=zeros(1,4);
% ss2_poses=zeros(1,4);
% for i=1:length(Actors)
%     ID=Actors(i).ActorID;
%     
%     if(ID==ss1_State(1))
%         ss1_poses=[Actors(i).Position(:)',ss1_State(1)];
%     elseif ID== (ss1_State(2))
%         ss2_poses=[Actors(i).Position(:)',ss1_State(2)];
%     
%     end
%   
% end
% ss1_poses(ss1_poses==0)=NaN;   
% ss2_poses(ss2_poses==0)=NaN;

== matlab function IntModelY1_20212r/Environment & Data/Visualisation & Data/Positions and States /MATLAB Function1 ==
  data: Actors input; TL_poses output; TL_State input

function TL_poses = findTLposes(Actors, TL_State)
n=length(TL_State);
TL_poses=zeros(n/2,5);
indices=zeros(n/2,1);
ID=zeros(length(Actors),1);

for i=1:length(Actors)
 ID(i)=Actors(i).ActorID;
end

indices=find(ismember(ID,TL_State(n/2+1:end)));
if (~isempty(indices))

    for i=1:n/2
        TL_poses(i,:)=([Actors(indices(i)).Position(:)',TL_State(i),ID(indices(i))]);

    end
end
TL_poses(TL_poses==0)=NaN;

== stateflow chart IntModelY1_20212r/Environment & Data/Visualisation & Data/Positions and States /Traffic Light Sensor/Traffic Light Switching Logic ==
  state STEADYRED
    entry:
    trafficLight(:)= Red; TL_ID=TL_id;
  state STEADYGREEN
    entry:
    trafficLight(:)= Green; TL_ID=TL_id;
  state START
    entry:
    trafficLight=TL_id;
    trafficLight(:)= Black;TL_ID=TL_id;
  state TRAFFICLIGHT_ODDYELLOW_EVENRED
    entry:
    trafficLight(1:2:end)=Yellow;TL_ID(1:2:end)=TL_id(1:2:end);
    trafficLight(2:2:end) = Red;TL_ID(2:2:end)=TL_id(2:2:end);
  state TRAFFICLIGHT_ODDGREEN_EVENRED
    entry:
    trafficLight(1:2:end)=Green;TL_ID(1:2:end)=TL_id(1:2:end);
    trafficLight(2:2:end) = Red;TL_ID(2:2:end)=TL_id(2:2:end);
  state TRAFFICLIGHT_ODDRED_EVENYELLOW
    entry:
    trafficLight(1:2:end)=Red;TL_ID(1:2:end)=TL_id(1:2:end);
    trafficLight(2:2:end) = Yellow;TL_ID(2:2:end)=TL_id(2:2:end);
  state TRAFFICLIGHT_ODDRED_EVENGREEN
    entry:
    trafficLight(1:2:end)=Red;TL_ID(1:2:end)=TL_id(1:2:end);
    trafficLight(2:2:end) = Green;TL_ID(2:2:end)=TL_id(2:2:end);
  (default) -> START
  START -> STEADYGREEN [order 3] : [LightConfig==1]
  START -> STEADYRED [order 1] : [LightConfig==2]
  START -> TRAFFICLIGHT_ODDGREEN_EVENRED [order 2] : [LightConfig ==3]
  TRAFFICLIGHT_ODDGREEN_EVENRED -> TRAFFICLIGHT_ODDYELLOW_EVENRED : after(4,sec)
  TRAFFICLIGHT_ODDYELLOW_EVENRED -> TRAFFICLIGHT_ODDRED_EVENGREEN : after(1,sec)
  TRAFFICLIGHT_ODDRED_EVENYELLOW -> TRAFFICLIGHT_ODDGREEN_EVENRED : after(1,sec)
  TRAFFICLIGHT_ODDRED_EVENGREEN -> TRAFFICLIGHT_ODDRED_EVENYELLOW : after(4,sec)
  data: Green constant double =3; Red constant double =1; Yellow constant double =2; LightConfig input; TL_id input; Black constant double =0; TL_ID output; trafficLight output

== matlab function IntModelY1_20212r/Environment & Data/Sensors & Perception/MATLAB Function ==
  data: SceneID output; ObjRelVel output; SceneRelVel output; SceneDist output; ObjectDist output; ObjAhead output; SDist input; Tracking input; SceneAhead output; RelVelmin output; RelDistmin output; Trans input
function [SceneID,ObjRelVel,SceneRelVel,SceneDist,ObjectDist,ObjAhead,SceneAhead,RelVelmin,RelDistmin]= SFDetections(SDist,Tracking, Trans)
ObjectID = zeros(20,1);
TrackPos = zeros(3,20);
TrackVel = zeros(3,20);
ObjectDist = 100; % zeros(20,1);
SceneDist = 100;
ObjRelVel = 10;
SceneRelVel = 10;
% ScenePos = [0 0];
ObjAhead = 0;
SceneAhead = 0;
SceneID = 0;
TracksNum = Tracking.NumTracks;

for t = 1:TracksNum
    ObjectID(t) = Tracking.Tracks(t).ObjectClassID;
    TrackPos(:,t) = Tracking.Tracks(t).State(1:2:5);
    TrackVel(:,t) = Tracking.Tracks(t).State(2:2:6);
   
    if TrackPos(2,t) < 1 && TrackPos(2,t) > -4 && abs(TrackPos(1,t)) <= SDist
        
        if ObjectID(t) >= 7 % 7=SS 8=TL 9=RA 10=RRC % labels {1,2,3,4} => {'TrafficLight','StopSign','RailRoadCrossing','RoundAbout'};
            SceneAhead = 1;
            SceneDist = min(SceneDist,TrackPos(1,t));
            if TrackPos(1,t) <= SceneDist
                % ScenePos = TrackPos(1:2,t)';
                SceneRelVel = TrackVel(1,t);
                SceneID = ObjectID(t);
            end
        end

        if ObjectID(t) < 7 && ObjectID(t) > 0
            ObjAhead = 1;
            ObjectDist = min(ObjectDist,TrackPos(1,t));
            if TrackPos(1,t) <= ObjectDist
                ObjRelVel = TrackVel(1,t);
                ObjID = ObjectID(t);
            end
        end

    end
    
end

if Trans == 1  % ObjectDist <= SceneDist
    RelVelmin = ObjRelVel;
    RelDistmin = ObjectDist;
else
    RelVelmin = min(SceneRelVel,ObjRelVel);
    RelDistmin = min(SceneDist,ObjectDist);
end

== matlab function IntModelY1_20212r/Vehicle Dynamics/Info2ActorState/MATLAB Function ==
  data: X input; Position output; Y input; Z input
function Position = fcn(X, Y, Z)

Position = [X Y, Z];
